simulink model "Vehicle_Dynamic_sim_V3_5"  (R2017a)
settings: Solver=FixedStepAuto  StartTime=0.0  StopTime=50  FixedStep=0.001  RelTol=1e-3  EnableMultiTasking=on
PreLoadFcn:
  | load ('CarSim_FE4_2.mat')
  | load ('Vehicle_information_test_0118_2017.mat')
values from neighbouring files (symbols this model uses):
  a = [(-2/tau - 1/tau_0) 1/tau 1/tau; 1/tau -2/tau 1/tau; 1/tau 1/tau -2/tau]    [MAE_272A_HW2_Q1a.m]    (also in Vehicle_Dynamic_main.m = 0.624; Vehicle_Dynamic_main_V0.m = 0.624; Vehicle_Dynamic_main_V01.m = 0.624; Vehicle_Dynamic_main_V0605.m = 0.624)
  aa = weight_front*wheelbase    (= 0.7875)    [Vehicle_Dynamic_main.m]    (also in Vehicle_Dynamic_main_V0.m; Vehicle_Dynamic_main_V01.m; Vehicle_Dynamic_main_V0605.m; Vehicle_Dynamic_main_V0629.m)
  b = [1/A 0; 0 1/A; 0 0]    [MAE_272A_HW2_Q1a.m]    (also in Vehicle_Dynamic_main.m = 0.624; Vehicle_Dynamic_main_V0.m = 0.624; Vehicle_Dynamic_main_V01.m = 0.624; Vehicle_Dynamic_main_V0605.m = 0.624)
  bb = weight_rear*wheelbase    (= 0.7875)    [Vehicle_Dynamic_main.m]    (also in Vehicle_Dynamic_main_V0.m; Vehicle_Dynamic_main_V01.m; Vehicle_Dynamic_main_V0605.m; Vehicle_Dynamic_main_V0629.m)
  g = 9.81    [Vehicle_Dynamic_main.m]    (also in Vehicle_Dynamic_main_V0.m; Vehicle_Dynamic_main_V01.m; Vehicle_Dynamic_main_V0605.m; Vehicle_Dynamic_main_V0629.m)
  hf = 0.20729    [Vehicle_Dynamic_main.m]    (also in Vehicle_Dynamic_main_V0.m; Vehicle_Dynamic_main_V01.m; Vehicle_Dynamic_main_V0605.m; Vehicle_Dynamic_main_V0629.m)
  hr = 0.20729    [Vehicle_Dynamic_main.m]    (also in Vehicle_Dynamic_main_V0.m; Vehicle_Dynamic_main_V01.m; Vehicle_Dynamic_main_V0605.m; Vehicle_Dynamic_main_V0629.m)
  initial_1 = [0 0 0 0]    [Vehicle_Dynamic_main.m]    (also in Vehicle_Dynamic_main_V0.m; Vehicle_Dynamic_main_V01.m; Vehicle_Dynamic_main_V0605.m; Vehicle_Dynamic_main_V0629.m)
  initial_2 = [0 0 0 0 (mf*g*weight_left/k_springf) (mf*g*weight_right/k_springf) ((mf*weight_left+mt)*g/k_tire_l) ((mf*weight_right+mt)*g/k_tire_r) 0]    [Vehicle_Dynamic_main.m]    (also in Vehicle_Dynamic_main_V0.m; Vehicle_Dynamic_main_V01.m; Vehicle_Dynamic_main_V0605.m; Vehicle_Dynamic_main_V0629.m)
  initial_3 = [0 0 0 0 (mr*g*weight_left/k_springr) (mr*g*weight_right/k_springr) ((mr*weight_left+mt)*g/k_tire_l) ((mr*weight_right+mt)*g/k_tire_r) 0]    [Vehicle_Dynamic_main.m]    (also in Vehicle_Dynamic_main_V0.m; Vehicle_Dynamic_main_V01.m; Vehicle_Dynamic_main_V0605.m; Vehicle_Dynamic_main_V0629.m)
  Izz = 89.99    [Vehicle_Dynamic_main.m]    (also in Vehicle_Dynamic_main_V0.m; Vehicle_Dynamic_main_V01.m; Vehicle_Dynamic_main_V0605.m; Vehicle_Dynamic_main_V0629.m)
  jf = mf*r_gy^2    (= 97.205445)    [Vehicle_Dynamic_main.m]    (also in Vehicle_Dynamic_main_V0.m; Vehicle_Dynamic_main_V01.m; Vehicle_Dynamic_main_V0605.m; Vehicle_Dynamic_main_V0629.m = 79.88796)
  jr = mr*r_gy^2    (= 97.205445)    [Vehicle_Dynamic_main.m]    (also in Vehicle_Dynamic_main_V0.m; Vehicle_Dynamic_main_V01.m; Vehicle_Dynamic_main_V0605.m; Vehicle_Dynamic_main_V0629.m = 79.88796)
  k_springf = 16640    [Vehicle_Dynamic_main.m]    (also in Vehicle_Dynamic_main_V0.m; Vehicle_Dynamic_main_V01.m; Vehicle_Dynamic_main_V0605.m; Vehicle_Dynamic_main_V0629.m = 13591.65)
  k_springr = 16640    [Vehicle_Dynamic_main.m]    (also in Vehicle_Dynamic_main_V0.m; Vehicle_Dynamic_main_V01.m; Vehicle_Dynamic_main_V0605.m; Vehicle_Dynamic_main_V0629.m = 13907.525)
  k_tire_l = 128571.4    [Vehicle_Dynamic_main.m]    (also in Vehicle_Dynamic_main_V0.m; Vehicle_Dynamic_main_V01.m; Vehicle_Dynamic_main_V0605.m; Vehicle_Dynamic_main_V0629.m)
  k_tire_r = 128571.4    [Vehicle_Dynamic_main.m]    (also in Vehicle_Dynamic_main_V0.m; Vehicle_Dynamic_main_V01.m; Vehicle_Dynamic_main_V0605.m; Vehicle_Dynamic_main_V0629.m)
  m_total = 237.6 + 70    (= 307.6)    [Vehicle_Dynamic_main.m]    (also in Vehicle_Dynamic_main_V0.m; Vehicle_Dynamic_main_V01.m; Vehicle_Dynamic_main_V0605.m; Vehicle_Dynamic_main_V0629.m = 252.8)
  mf = m_total*weight_front    (= 153.8)    [Vehicle_Dynamic_main.m]    (also in Vehicle_Dynamic_main_V0.m; Vehicle_Dynamic_main_V01.m; Vehicle_Dynamic_main_V0605.m; Vehicle_Dynamic_main_V0629.m = 126.4)
  mr = m_total*weight_rear    (= 153.8)    [Vehicle_Dynamic_main.m]    (also in Vehicle_Dynamic_main_V0.m; Vehicle_Dynamic_main_V01.m; Vehicle_Dynamic_main_V0605.m; Vehicle_Dynamic_main_V0629.m = 126.4)
  mt = 27.4/2    (= 13.7)    [Vehicle_Dynamic_main.m]    (also in Vehicle_Dynamic_main_V0.m; Vehicle_Dynamic_main_V01.m; Vehicle_Dynamic_main_V0605.m; Vehicle_Dynamic_main_V0629.m)
  r_damperf = 1416.7    [Vehicle_Dynamic_main.m]    (also in Vehicle_Dynamic_main_V0.m; Vehicle_Dynamic_main_V01.m; Vehicle_Dynamic_main_V0605.m; Vehicle_Dynamic_main_V0629.m = 5000)
  r_damperr = 1416.7    [Vehicle_Dynamic_main.m]    (also in Vehicle_Dynamic_main_V0.m; Vehicle_Dynamic_main_V01.m; Vehicle_Dynamic_main_V0605.m; Vehicle_Dynamic_main_V0629.m = 1428.6)
  sp_max = 30    [Vehicle_Dynamic_main.m]    (also in Vehicle_Dynamic_main_V0.m; Vehicle_Dynamic_main_V01.m; Vehicle_Dynamic_main_V0605.m; Vehicle_Dynamic_main_V0629.m)
  Tire_data_1 = [0	10.16645	30.135844	49.972681	69.612462	88.995136	108.063766	126.765417	145.053829	162.887632	180.230352	197.053076	213.331781	229.048232	244.189973	258.748997	272.722636	286.111778	298.921762	311.160594	322.839396	333.970622	344.56984	354.653955	364.239424	373.34582	381.991381	390.195233	397.976949	405.355211	412.349148	418.976995	425.256992	431.206487	436.841937	442.179356	447.234758	452.02326 ...(+3067 chars)    [Vehicle_Dynamic_main.m]    (also in Vehicle_Dynamic_main_V0.m; Vehicle_Dynamic_main_V01.m; Vehicle_Dynamic_main_V0605.m; Vehicle_Dynamic_main_V0629.m)
  track = 1.248    [Vehicle_Dynamic_main.m]    (also in Vehicle_Dynamic_main_V0.m; Vehicle_Dynamic_main_V01.m; Vehicle_Dynamic_main_V0605.m; Vehicle_Dynamic_main_V0629.m)
(part 3 of 3)

== matlab function Vehicle_Dynamic_sim_V3_5/SubVehicle Dynamic Model (Linear Damper): FE4/Subsystem1/MATLAB Function ==
  data: t input; ds output; s2 input; Fcl_r input; Fcr_r input; Vroad_left_r input; Vroad_right_r input; ext output; mr parameter; g parameter; jr parameter; a parameter; b parameter; k_springr parameter; r_damperr parameter; k_tire_l parameter; k_tire_r parameter; hr parameter; mt parameter; Fs input
function [ds,ext] = weight_tr_rear_fcn(t,s2,Fcl_r,Fcr_r,Vroad_left_r,Vroad_right_r,mr, g, jr, a, b, k_springr, r_damperr, k_tire_l, k_tire_r, hr, mt, Fs)

%global m g j a b k_springf r_damperf k_tire_l k_tire_r F h mt 

% state variables
Pjr = s2(1); %roll momentum of sprung mass
Pvr = s2(2); %heave momentum of sprung mass
Ptlr = s2(3); %momentum of tire at left
Ptrr = s2(4); %momentum of tire at right
qslr = s2(5); %displacement of spring at left
qsrr = s2(6); %displacement of spring at right
qsltr = s2(7); %displacement of tire at left
qsrtr = s2(8); %displacement of tire at right
roll_angler = s2(9); %Roll angle

%Lateral acceleration input

if qsltr < 0
    k_tire_l_s = 0;
else
    k_tire_l_s = k_tire_l;
end

if qsrtr < 0
    k_tire_r_s = 0;
else
    k_tire_r_s = k_tire_r;
end


%State variable
dPj = (-(r_damperr/jr)*(b^2+a^2))*Pjr + ((r_damperr/mr)*(b-a))*Pvr - ((b*r_damperr)/mt)*Ptlr + ((a*r_damperr/mt))*Ptrr + b*k_springr*qslr - a*k_springr*qsrr + Fs*hr*cos(roll_angler) + mr*g*sin(roll_angler) + b*Fcl_r - a*Fcr_r;
      
dPv = (r_damperr/jr)*(b-a)*Pjr - (2*r_damperr/mr)*Pvr + (r_damperr/mt)*Ptlr + (r_damperr/mt)*Ptrr - k_springr*qslr - k_springr*qsrr - Fcl_r - Fcr_r + mr*g;
      
dPtl = (-b*r_damperr/jr)*Pjr + (r_damperr/mr)*Pvr - (r_damperr/mt)*Ptlr + k_springr*qslr - k_tire_l_s*qsltr + Fcl_r + mt*g;
     
dPtr = (a*r_damperr/jr)*Pjr + (r_damperr/mr)*Pvr - (r_damperr/mt)*Ptrr + k_springr*qsrr - k_tire_r_s*qsrtr + Fcr_r + mt*g;
      
dqsl = (-b/jr)*Pjr + (1/mr)*Pvr - (1/mr)*Ptlr;

dqsr = (a/jr)*Pjr + (1/mr)*Pvr - (1/mr)*Ptrr;

dqslt = (1/mt)*Ptlr - Vroad_left_r;

dqsrt = (1/mt)*Ptrr - Vroad_right_r;

droll_angle = Pjr/jr;

%Output
force_input = Fs;

force_on_lefttire_front = k_tire_l_s*qsltr;

force_on_righttire_front = k_tire_r_s*qsrtr;

roll_angular_speed_front = Pjr/jr;

ds = [dPj;dPv;dPtl;dPtr;dqsl;dqsr;dqslt;dqsrt;droll_angle];
ext = [force_input;force_on_lefttire_front;force_on_righttire_front;roll_angular_speed_front];

== matlab function Vehicle_Dynamic_sim_V3_5/SubVehicle Dynamic Model (Linear Damper): FE1/MATLAB Function ==
  data: ds output; s input; theta input; t input; Fr input; Fl input; Fyf input; Fyr input; u input; ext output; aa parameter; bb parameter; m_total parameter; Izz parameter; track parameter; delta input
function [ds, ext] = vehicle_dyanmic_fun(s,theta,t,Fr,Fl,Fyf,Fyr,u, aa, bb, m_total, Izz, track, delta)

% state variables
Py = s(1); %Lateral linear momentum
Pr = s(2); %Yaw angula momentum 
Lx = s(3); %Position on X-axis
Ly = s(4); %Position on Y-axis

dPy = Fyf*cos(delta) + Fyr - (m_total*u/Izz)*Pr;
dPr = aa*Fyf*cos(delta) - bb*Fyr + 0.5*track*Fr - 0.5*track*Fl;
dLx = u*cos(theta)-(Py/m_total)*sin(theta);
dLy = (Py/m_total*cos(theta)) + (u*sin(theta));

yaw_rate = Pr/Izz;
X_out = Lx;
Y_out = Ly;



ext = [yaw_rate;X_out;Y_out];
ds = [dPy;dPr;dLx;dLy];

== matlab function Vehicle_Dynamic_sim_V3_5/SubVehicle Dynamic Model (Linear Damper): FE1/MATLAB Function1 ==
  data: Py input; Pr input; delta_l input; delta_r input; alphaf_l output; u input; alphaf_r output; alphar_l output; alphar_r output; aa parameter; bb parameter; Izz parameter; m_total parameter; delta_avg output
function [alphaf_l,alphaf_r,alphar_l,alphar_r,delta_avg] = slip_angle_fcn(Py,Pr,delta_l, delta_r,u, aa, bb, Izz, m_total)
%#codegen

wy = Pr/Izz;
v = Py/m_total;

alphaf_l = (delta_l*pi/180) - atan2((v+aa*wy),u);
alphaf_r = (delta_r*pi/180) - atan2((v+aa*wy),u);
alphar_l = -atan2((v-bb*wy),u);
alphar_r = -atan2((v-bb*wy),u);

delta_avg = 0.5*(delta_l+delta_r)*pi/180;
end

== matlab function Vehicle_Dynamic_sim_V3_5/SubVehicle Dynamic Model (Linear Damper): FE1/MATLAB Function3 ==
  data: force_on_lefttire_rear output; ay input; force_on_righttire_rear output; mr parameter; g parameter; a parameter; b parameter; hf parameter; mt parameter
function [force_on_lefttire_rear,force_on_righttire_rear] = weight_tr_rear_fcn(ay, mr, g, a, b, hf,mt)
%#codegen
m=mr+2*mt;
diff_weight_tr = ay*hf/(a+b)*m;

force_on_lefttire_rear = (0.5*m-diff_weight_tr)*g;
force_on_righttire_rear = (0.5*m+diff_weight_tr)*g;

== matlab function Vehicle_Dynamic_sim_V3_5/Desired Yaw Rate ==
  data: u input; yaw_desire output; steer_angle input; aa parameter; bb parameter
function yaw_desire = fcn(u,steer_angle, aa, bb)


yaw_desire = u*steer_angle*pi/180/(aa+bb);

== matlab function Vehicle_Dynamic_sim_V3_5/SubVehicle Dynamic Model (Linear Damper): FE1/MATLAB Function2 ==
  data: force_on_lefttire_front output; ay input; force_on_righttire_front output; mf parameter; g parameter; a parameter; b parameter; hf parameter; mt parameter
function [force_on_lefttire_front,force_on_righttire_front] = weight_tr_front_fcn(ay, mf, g, a, b, hf,mt)
%#codegen

m=mf+2*mt;
diff_weight_tr = ay*hf/(a+b)*m;

force_on_lefttire_front = (0.5*m-diff_weight_tr)*g;
force_on_righttire_front = (0.5*m+diff_weight_tr)*g;
